simulink model "Q1"  (R2020a)
settings: Solver=FixedStepAuto  StartTime=0.0  StopTime=0.06  FixedStep=1e-05  RelTol=1e-3
libraries: powerlib x14, powerlib_meascontrol x1
settings Model: Creator=furka  LastModifiedBy=Baris Emektar
settings SFSimCC: CustomCodeUndefinedFunction=UseInterfaceOnly

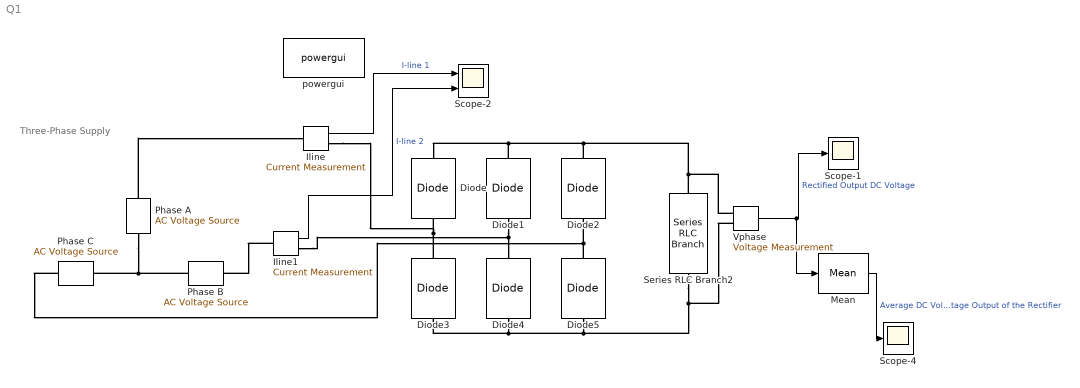
== system Q1 ==
  note: Three-Phase Supply
  Diode{,1..5} (6 alike) : powerlib/Power Electronics/Diode  Ron=0  Lon=0  Vf=0  IC=0  UseSnubber=0  Rs=0  Cs=0  Measurements=off
  Iline : powerlib/Measurements/Current Measurement  PhasorSimulation=off  OutputType=Complex  PSBequivalent=0
  Iline1 : powerlib/Measurements/Current Measurement  PhasorSimulation=off  OutputType=Complex  PSBequivalent=0
  Mean : powerlib_meascontrol/Measurements/Mean  Freq=60  Vinit=0  Ts=0
  Phase A : powerlib/Electrical Sources/AC Voltage Source  Amplitude=400*sqrt(2)/sqrt(3)  Phase=0  Frequency=50  SampleTime=0  Measurements=None  BusType=swing  Pref=10e3  Qref=0  Qmin=-inf  Qmax=+inf
  Phase B : powerlib/Electrical Sources/AC Voltage Source  Amplitude=400*sqrt(2)/sqrt(3)  Phase=120  Frequency=50  SampleTime=0  Measurements=None  BusType=swing  Pref=10e3  Qref=0  Qmin=-inf  Qmax=+inf
  Phase C : powerlib/Electrical Sources/AC Voltage Source  Amplitude=400*sqrt(2)/sqrt(3)  Phase=240  Frequency=50  SampleTime=0  Measurements=None  BusType=swing  Pref=10e3  Qref=0  Qmin=-inf  Qmax=+inf
  Scope-1 : Scope
  Scope-2 : Scope  NumInputPorts=2
  Scope-4 : Scope
  Series RLC Branch2 : powerlib/Elements/Series RLC Branch  LConnTagsString=__new0  RConnTagsString=__new0  BranchType=R  Resistance=97.2  Inductance=0  SetiL0=off  InitialCurrent=0  Capacitance=1e-6  Setx0=off  InitialVoltage=0  Measurements=None
  Vphase : powerlib/Measurements/Voltage Measurement  PhasorSimulation=off  OutputType=Complex  PSBequivalent=0
  powergui : powerlib/powergui  Priority=1  SimulationMode=Continuous  SampleTime=1e-5  frequency=60  Iterations=50  frequencyindice=50  Pbase=100e6  ErrMax=1e-4  UnitsV=kV  UnitsW=MW  buscounter=0  FunctionMessages=off  echomessages=off  EnableUseOfTLC=off  CurrentSourceSwitches=off  DisableSnubberDevices=off  DisableRonSwitches=off  DisableVfSwitches=off  DisplayEquations=off  AutomaticDiscreteSolvers=off  SolverType=Tustin/Backward Euler (TBE)  Interpol=off  ExternalGateDelay=off  methode=off  Ts=100  x0status=blocks  SPID=on  SwTol=0  HookPort=off  NonlinearTolerance=0  nMaxIteration=15  ContinueOnMaxIteration=off  RestoreLinks=warning  ResistiveCurrentMeasurement=off  Frange=[0:2:500]  Ylog=off  Xlog=on  ShowGrid=off  save=off  variable=ZData  structure=0  ZoomFFT=off  StartTime=0.0  cycles=1  DisplayStyle=1  fundamental=60  FreqAxis=off  MaxFrequency=1000  frequencyindicesteady=1  RmsSteady=1  display=off
  wires:
  Vphase/1 -> Mean/1, Scope-1/1  "Rectified Output DC Voltage"
  Iline/1 -> Scope-2/1  "I-line 1"
  Iline1/1 -> Scope-2/2  "I-line 2"
  Mean/1 -> Scope-4/1  "Average DC Voltage Output of the Rectifier"
  connections:
  Phase B/LConn1 -- Phase A/LConn1 -- Phase C/LConn1
  Phase A/RConn1 -- Iline/LConn1
  Diode3/RConn1 -- Iline/RConn1 -- Diode/LConn1
  Diode1/LConn1 -- Iline1/RConn1 -- Diode4/RConn1
  Diode5/RConn1 -- Phase C/RConn1 -- Diode2/LConn1
  Series RLC Branch2/RConn1 -- Vphase/LConn1 -- Diode2/RConn1 -- Diode1/RConn1 -- Diode/RConn1
  Series RLC Branch2/LConn1 -- Vphase/LConn2 -- Diode5/LConn1 -- Diode4/LConn1 -- Diode3/LConn1
  Iline1/LConn1 -- Phase B/RConn1
